simulink model "Amplifier"  (R2023a)
settings: Solver=VariableStepAuto  StartTime=0.0  StopTime=10  RelTol=1e-3
model workspace (MAT data in the model file):
  R1 = 20
  R2 = 500
  VT = 0.5
  a = 500
  b = 1000
settings Model: Creator=Wang Xishengshun  LastModifiedBy=Wang Xishengshun

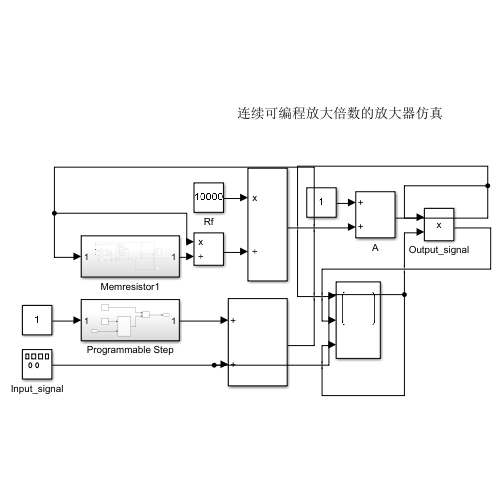
[thumbnail: Simulink's stored preview of the top-level diagram]
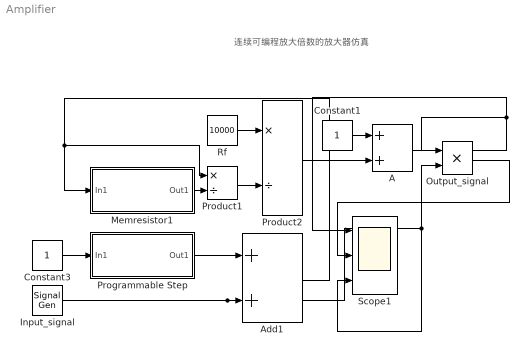
== system Amplifier ==
  note: 连续可编程放大倍数的放大器仿真
  A : Sum
  Add1 : Sum
  Constant1 : Constant
  Constant3 : Constant
  Input_signal : SignalGenerator  Frequency=10  Units=rad/sec
  Memresistor1 : Subsystem
  Output_signal : Product
  Product1 : Product  Inputs=*/
  Product2 : Product  Inputs=*/
  Programmable Step : Subsystem
  Rf : Constant  Value=10000
  Scope1 : Scope  NumInputPorts=3
  wires:
  Memresistor1/1(Out1) -> Product1/2
  Product1/1 -> Product2/2
  Rf/1 -> Product2/1
  Constant1/1 -> A/1
  A/1 -> Output_signal/1, Scope1/1
  Output_signal/1 -> Scope1/2
  Constant3/1 -> Programmable Step/1(In1)
  Input_signal/1 -> Scope1/3, Output_signal/2, Add1/2
  Programmable Step/1(Out1) -> Add1/1
  Add1/1 -> Memresistor1/1(In1), Product1/1
  Product2/1 -> A/2

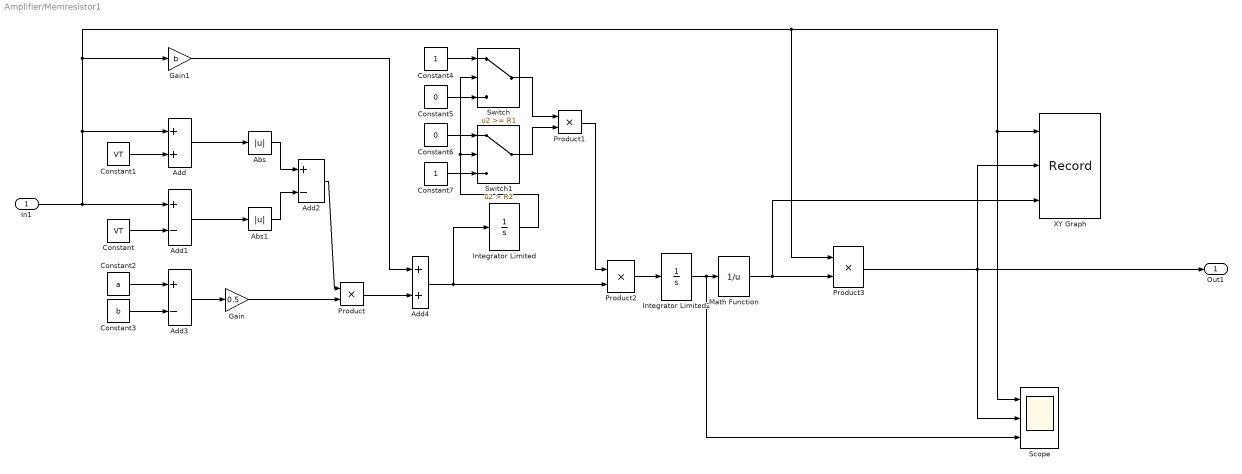
== system Amplifier/Memresistor1 ==
  In1 : Inport
  Abs : Abs  SaturateOnIntegerOverflow=off
  Abs1 : Abs  SaturateOnIntegerOverflow=off
  Add : Sum
  Add1 : Sum  Inputs=+-
  Add2 : Sum  Inputs=+-
  Add3 : Sum  Inputs=+-
  Add4 : Sum
  Constant : Constant  Value=VT
  Constant1 : Constant  Value=VT
  Constant2 : Constant  Value=a
  Constant3 : Constant  Value=b
  Constant4 : Constant  SampleTime=0.001
  Constant5 : Constant  Value=0  SampleTime=0.001
  Constant6 : Constant  Value=0  SampleTime=0.001
  Constant7 : Constant  SampleTime=0.001
  Gain : Gain  Gain=0.5
  Gain1 : Gain  Gain=b
  Integrator Limited : Integrator  UpperSaturationLimit=1600  LowerSaturationLimit=0  WrappedStateUpperValue=500  WrappedStateLowerValue=0
  Integrator Limited2 : Integrator  InitialCondition=480  UpperSaturationLimit=1600  LowerSaturationLimit=0  WrappedStateUpperValue=500  WrappedStateLowerValue=0
  Math Function : Math  Operator=reciprocal
  Product{,1..3} (4 alike) : Product
  Scope : Scope  NumInputPorts=3
  Switch : Switch  Threshold=R1  RndMeth=Ceiling  SaturateOnIntegerOverflow=off  InputSameDT=off
  Switch1 : Switch  Criteria=u2 > Threshold  Threshold=R2  RndMeth=Ceiling  SaturateOnIntegerOverflow=off  InputSameDT=off
  XY Graph : Record  FileSettingsInternal="{\"entries\":[{\"content\":{\"excelSettings\":{\"content\":{},\"type\":\"Streamout.ExcelSettings\"}},\"type\":\"Streamout.FileSettingStorage\",\"uuid\":\"\"}],\"packageUris\":[\"http:\\/\\/schema.mathworks.com\\/mf0\\/streamout_blocks\\/R2020a\"],\"version\":\"1.0\"}"  Layout=[2 2]  SignalsInternal="{\"entries\":[{\"content\":{\"signals\":[{\"content\":{\"blockPath\":[],\"dimensions\":[1],\"domain\":\"\",\"lineColor\":\"#a2142f\",\"plots\":[1,9],\"port\":1,\"sid\":[\"\"],\"signalID\":22,\"signalName\":\"In1\"},\"type\":\"RecordBlkView.Signal\",\"uuid\":\"\"},{\"content\":{\"blockPath\":[],\"dimensions\":[1],\"domain\":\"\",\"lineColor\":\"#139fff\",\"plots\":[9],\"port\":2,\"sid\":[\"\"],\"signalID\":26,\"signalName\":\"Product3\"},\"type\":\"RecordBlkView.Signal\",\"uuid\":\"\"},{\"content\":{\"blockPath\":[],\"dimensions\":[1],\"domain\":\"\",\"lineColor\":\"#77ac30\",\"plots\":[1],\"port\":3,\"sid\":[\"\"],\"signalID\":30,\"signalName\":\"Math\\nFunction\"},\"type\":\"RecordBlkView.Signal\",\"uuid\":\"\"}]},\"type\":\"RecordBlkView.InputSignals\",\"uuid\":\"\"}],\"packageUris\":[\"http:\\/\\/schema.mathworks.com\\/mf0\\/streamout_blocks\\/R2020a\"],\"version\":\"1.0\"}"  VisualizationBindings="{\"xyplotplugin\":{\"info\":[{\"series\":[{\"bindingParametersList\":[{\"parameter\":\"X-Axis\",\"signalID\":30,\"signalName\":\"Math\\nFunction\"}],\"seriesID\":48},{\"bindingParametersList\":[{\"parameter\":\"X-Axis\",\"signalID\":22,\"signalName\":\"In1\"},{\"parameter\":\"Y-Axis\",\"signalID\":30,\"signalName\":\"Math\\nFunction\"}],\"seriesID\":25716}],\"subplotID\":1},{\"series\":[{\"bindingParametersList\":[{\"parameter\":\"X-Axis\",\"signalID\":22,\"signalName\":\"In1\"},{\"parameter\":\"Y-Axis\",\"signalID\":26,\"signalName\":\"Product3\"}],\"seriesID\":21706}],\"subplotID\":9}]}}"  CompatibilityTag=XY
  Out1 : Outport
  wires:
  Product3/1 -> Scope/2, Out1/1, XY Graph/2
  Constant2/1 -> Add3/1
  Product/1 -> Add4/2
  Integrator Limited/1 -> Switch/2, Switch1/2
  Product1/1 -> Product2/1
  Add/1 -> Abs/1
  Math Function/1 -> XY Graph/3, Product3/2
  Gain1/1 -> Add4/1
  Constant7/1 -> Switch1/3
  Constant3/1 -> Add3/2
  Add1/1 -> Abs1/1
  Switch/1 -> Product1/1
  Constant6/1 -> Switch1/1
  Constant5/1 -> Switch/3
  Abs/1 -> Add2/1
  Switch1/1 -> Product1/2
  Product2/1 -> Integrator Limited2/1
  Gain/1 -> Product/2
  Add2/1 -> Product/1
  Constant1/1 -> Add/2
  Constant4/1 -> Switch/1
  Add4/1 -> Integrator Limited/1, Product2/2
  In1/1 -> Add1/1, Scope/1, XY Graph/1, Product3/1, Gain1/1, Add/1
  Integrator Limited2/1 -> Scope/3, Math Function/1
  Abs1/1 -> Add2/2
  Constant/1 -> Add1/2
  Add3/1 -> Gain/1

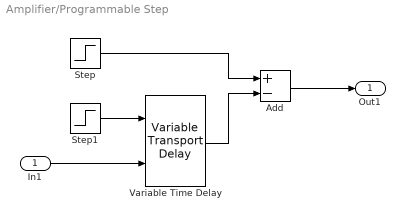
== system Amplifier/Programmable Step ==
  In1 : Inport
  Add : Sum  Inputs=+-
  Step : Step  Time=0  SampleTime=0
  Step1 : Step  Time=0  SampleTime=0
  Variable Time Delay : VariableTransportDelay  MaximumDelay=10
  Out1 : Outport
  wires:
  Step1/1 -> Variable Time Delay/1
  In1/1 -> Variable Time Delay/2
  Variable Time Delay/1 -> Add/2
  Step/1 -> Add/1
  Add/1 -> Out1/1
